simulink model "nbus_dyna_angle_change_II"  (R2023a)
settings: Solver=VariableStepAuto  StartTime=0.0  StopTime=100  RelTol=1e-3
values from neighbouring files (symbols this model uses):
  Load = 1.4062    [ee5802.m]
  rpu = R/Rbase    [ee5802.m]
settings Model: Creator=Jecordjo  LastModifiedBy=Jecordjo

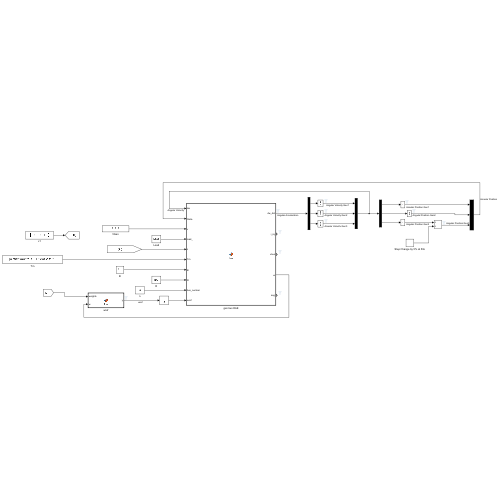
[thumbnail: Simulink's stored preview of the top-level diagram]
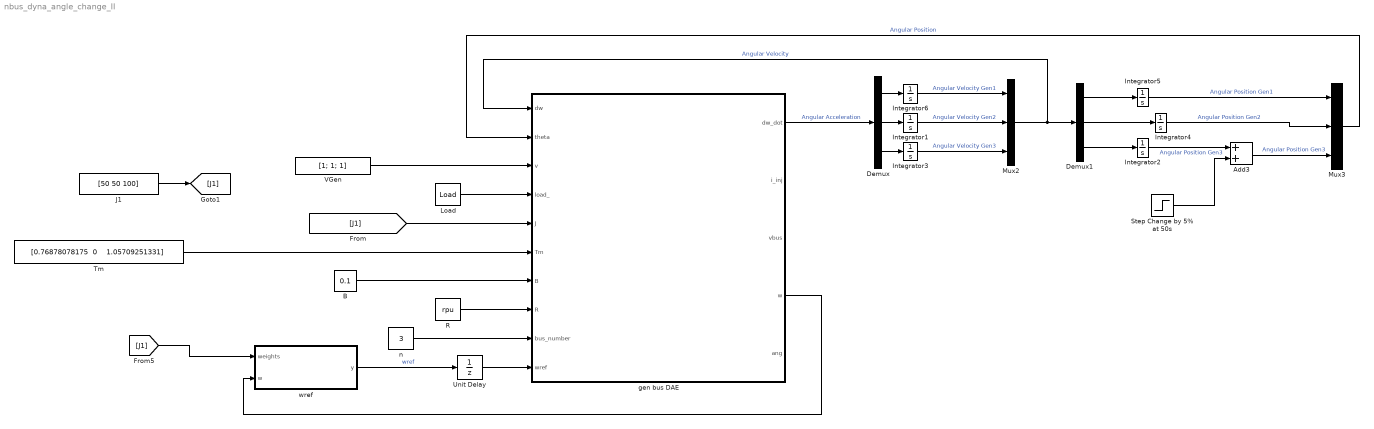
== system nbus_dyna_angle_change_II ==
  Add3 : Sum
  B : Constant  Value=0.1
  Demux : Demux  Outputs=3
  Demux1 : Demux  Outputs=3
  Integrator{1,3,5..6} (4 alike) : Integrator
  Integrator2 : Integrator  InitialCondition=0.1019
  Integrator4 : Integrator  InitialCondition=0.2385668530558521
  J1 : Constant  Value=[50 50 100]
  Load : Constant  Value=Load
  Mux2 : Mux  Inputs=3
  Mux3 : Mux  Inputs=3
  R : Constant  Value=rpu
  Step Change by 5% at 50s : Step  Time=50  After=0.005  SampleTime=0
  Tm : Constant  Value="[0.76878078175  0    1.05709251331]"
  Unit Delay : UnitDelay  InitialCondition=1  SampleTime=-1  HasFrameUpgradeWarning=on
  VGen : Constant  Value=[1; 1; 1]
  gen bus DAE : MATLAB Function  TreatAsAtomicUnit=on
  n : Constant  Value=3
  wref : MATLAB Function  TreatAsAtomicUnit=on
  wires:
  Demux/1 -> Integrator6/1
  Integrator6/1 -> Mux2/1  "Angular Velocity Gen1"
  Add3/1 -> Mux3/3  "Angular Position Gen3"
  [J1] -> wref/1(weights)
  Integrator2/1 -> Add3/1  "Angular Position Gen3"
  B/1 -> gen bus DAE/7(B)
  Integrator3/1 -> Mux2/3  "Angular Velocity Gen3"
  Demux1/3 -> Integrator2/1
  Integrator4/1 -> Mux3/2  "Angular Position Gen2"
  Step Change by 5% at 50s/1 -> Add3/2
  Mux3/1 -> gen bus DAE/2(theta)  "Angular Position"
  Demux/3 -> Integrator3/1
  J1/1 -> [J1]
  wref/1(y) -> Unit Delay/1  "wref"
  Integrator1/1 -> Mux2/2  "Angular Velocity Gen2"
  Demux1/1 -> Integrator5/1
  R/1 -> gen bus DAE/8(R)
  gen bus DAE/4(w) -> wref/2(w)
  Demux1/2 -> Integrator4/1
  Tm/1 -> gen bus DAE/6(Tm)
  VGen/1 -> gen bus DAE/3(v)
  Load/1 -> gen bus DAE/4(load_)
  Integrator5/1 -> Mux3/1  "Angular Position Gen1"
  Mux2/1 -> Demux1/1, gen bus DAE/1(dw)  "Angular Velocity"
  Demux/2 -> Integrator1/1
  gen bus DAE/1(dw_dot) -> Demux/1  "Angular Acceleration"
  n/1 -> gen bus DAE/9(bus_number)
  Unit Delay/1 -> gen bus DAE/10(wref)
  [J1] -> gen bus DAE/5(J)

== matlab function nbus_dyna_angle_change_II/gen bus DAE ==
  data: dw input; theta input size=3; dw_dot output size=3; i_inj output size=3; v input size=3; load_ input; J input; Tm input; B input; vbus output; R input; bus_number input; wref input; w output; ang output
function [dw_dot, i_inj , vbus, w, ang] = fcn(dw,theta,v,load_,J,Tm,B,R,bus_number,wref)
n=bus_number;
% x0 = zeros(2,n);
w=zeros(3,1);
dw_dot = zeros(3,1);
ang=[0 0 0];
% x0(2,1) = load_(1);
% for j = 2:n
%     x0(1,j) = v(1);
%     x0(2,j) = load_(j);
% end
w=dw+[wref;wref;wref];
x0 = [v(1) v(2) v(3);1.05 0 1.01;theta(1) theta(2) theta(3)];
sol = fsolve(@(x) solving_systems_nbus(x, [v(1) v(2) v(3)], [-1 0 -1], load_, R, n, [theta(1) -1 theta(3)]),x0,optimoptions('fsolve','Display','off','Algorithm','levenberg-marquardt'));

i_inj = sol(2,:)';

vbus = sol(1,:);

ang = sol(3,:);

dw_dot(1) = (1/J(1))*(Tm(1) - ((v(1)*i_inj(1)*cos(sol(3,1)))/w(1)) - B*w(1) - 100*dw(1));
dw_dot(2) = 0;
dw_dot(3) =  (1/J(3))*(Tm(3) - ((v(3)*i_inj(3)*cos(sol(3,3)))/w(3)) - B*w(3) - 100*dw(3));

== matlab function nbus_dyna_angle_change_II/wref ==
  data: weights input; w input; y output
function y = fcn(weights,w)
    
y = sum(w.*(weights/sum(weights)));
